simulink library "TESTSEN4CH"  (Simulink 8.5)
settings: Solver=ode45  StartTime=0.0  StopTime=10.0  RelTol=1e-3
libraries: cdsFilt x4, VIS_LIB x2, cdsFunctionCall x1
settings Model: Creator=controls  LastModifiedBy=controls

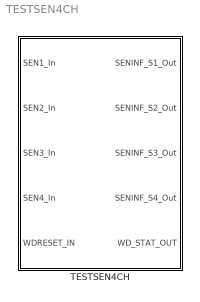
== system TESTSEN4CH ==
  TESTSEN4CH : Subsystem

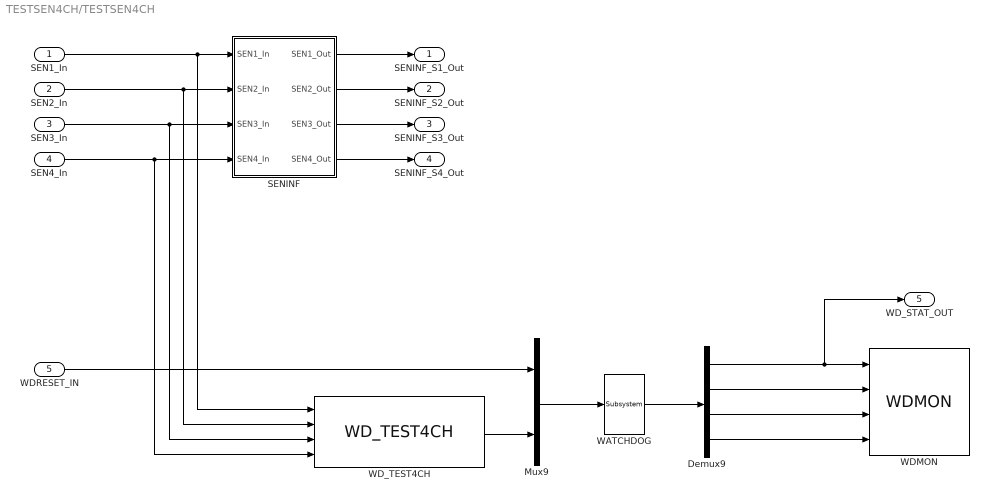
== system TESTSEN4CH/TESTSEN4CH ==
  SEN1_In : Inport
  SEN2_In : Inport  Port=2
  SEN3_In : Inport  Port=3
  SEN4_In : Inport  Port=4
  WDRESET_IN : Inport  Port=5
  Demux9 : Demux
  Mux9 : Mux  Inputs=2
  SENINF : Subsystem
  WATCHDOG : cdsFunctionCall/Subsystem  Tag=cdsFunctionCall  Description=inline OSEMWATCHDOG /opt/rtcds/userapps/release/vis/common/src/WATCHDOG.c
      settings: AttributesFormatString=%<Tag>\n%<Description>
  WDMON : VIS_LIB/WDMON
  WD_TEST4CH : VIS_LIB/WD_TEST4CH
  SENINF_S1_Out : Outport
  SENINF_S2_Out : Outport  Port=2
  SENINF_S3_Out : Outport  Port=3
  SENINF_S4_Out : Outport  Port=4
  WD_STAT_OUT : Outport  Port=5
  wires:
  Demux9/2 -> WDMON/2
  Demux9/3 -> WDMON/3
  WD_TEST4CH/1 -> Mux9/2
  WATCHDOG/1 -> Demux9/1
  Demux9/4 -> WDMON/4
  Mux9/1 -> WATCHDOG/1
  Demux9/1 -> WD_STAT_OUT/1, WDMON/1
  SEN1_In/1 -> WD_TEST4CH/1, SENINF/1(SEN1_In)
  WDRESET_IN/1 -> Mux9/1
  SEN2_In/1 -> WD_TEST4CH/2, SENINF/2(SEN2_In)
  SEN3_In/1 -> WD_TEST4CH/3, SENINF/3(SEN3_In)
  SEN4_In/1 -> WD_TEST4CH/4, SENINF/4(SEN4_In)
  SENINF/1(SEN1_Out) -> SENINF_S1_Out/1
  SENINF/2(SEN2_Out) -> SENINF_S2_Out/1
  SENINF/3(SEN3_Out) -> SENINF_S3_Out/1
  SENINF/4(SEN4_Out) -> SENINF_S4_Out/1

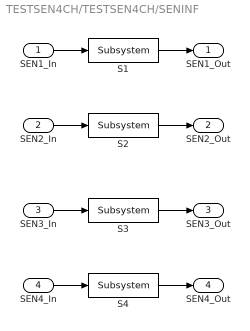
== system TESTSEN4CH/TESTSEN4CH/SENINF ==
  SEN1_In : Inport
  SEN2_In : Inport  Port=2
  SEN3_In : Inport  Port=3
  SEN4_In : Inport  Port=4
  S1 : cdsFilt/Subsystem  Tag=cdsFilt  Description=|
      | Purpose:                                                                                                                                                                                                                                  
      | Standard CDS IIR filter module.                                                                                                                                                                                                           
      |                                                                                                                                                                                                                                           
      | Operation:                                                                                                                                                                                                                                
      | Consists of 10 second order section IIR filters, plus a ramped gain stage. In FE code, also provides pre-defined test points and excitation channel inputs. The filter coefficients are defined in the LIGO system using the 'foton' tool.
      |                                                                                                                                                                                                                                           
      | Usage:                                                                                                                                                                                                                                    
      | Name the part with the desired filter module name.
      settings: AttributesFormatString=%<Tag>
  S2 : cdsFilt/Subsystem  Tag=cdsFilt  Description=|
      | Purpose:                                                                                                                                                                                                                                  
      | Standard CDS IIR filter module.                                                                                                                                                                                                           
      |                                                                                                                                                                                                                                           
      | Operation:                                                                                                                                                                                                                                
      | Consists of 10 second order section IIR filters, plus a ramped gain stage. In FE code, also provides pre-defined test points and excitation channel inputs. The filter coefficients are defined in the LIGO system using the 'foton' tool.
      |                                                                                                                                                                                                                                           
      | Usage:                                                                                                                                                                                                                                    
      | Name the part with the desired filter module name.
      settings: AttributesFormatString=%<Tag>
  S3 : cdsFilt/Subsystem  Tag=cdsFilt  Description=|
      | Purpose:                                                                                                                                                                                                                                  
      | Standard CDS IIR filter module.                                                                                                                                                                                                           
      |                                                                                                                                                                                                                                           
      | Operation:                                                                                                                                                                                                                                
      | Consists of 10 second order section IIR filters, plus a ramped gain stage. In FE code, also provides pre-defined test points and excitation channel inputs. The filter coefficients are defined in the LIGO system using the 'foton' tool.
      |                                                                                                                                                                                                                                           
      | Usage:                                                                                                                                                                                                                                    
      | Name the part with the desired filter module name.
      settings: AttributesFormatString=%<Tag>
  S4 : cdsFilt/Subsystem  Tag=cdsFilt  Description=|
      | Purpose:                                                                                                                                                                                                                                  
      | Standard CDS IIR filter module.                                                                                                                                                                                                           
      |                                                                                                                                                                                                                                           
      | Operation:                                                                                                                                                                                                                                
      | Consists of 10 second order section IIR filters, plus a ramped gain stage. In FE code, also provides pre-defined test points and excitation channel inputs. The filter coefficients are defined in the LIGO system using the 'foton' tool.
      |                                                                                                                                                                                                                                           
      | Usage:                                                                                                                                                                                                                                    
      | Name the part with the desired filter module name.
      settings: AttributesFormatString=%<Tag>
  SEN1_Out : Outport
  SEN2_Out : Outport  Port=2
  SEN3_Out : Outport  Port=3
  SEN4_Out : Outport  Port=4
  wires:
  S1/1 -> SEN1_Out/1
  SEN1_In/1 -> S1/1
  S2/1 -> SEN2_Out/1
  SEN2_In/1 -> S2/1
  S3/1 -> SEN3_Out/1
  SEN3_In/1 -> S3/1
  S4/1 -> SEN4_Out/1
  SEN4_In/1 -> S4/1
